simulink model "MBR_2025_09_29_Wassertank_nichtlinear_linear"  (R2024b)
settings: Solver=VariableStepAuto  StartTime=0.0  StopTime=10  RelTol=1e-3
settings Model: Creator=raroth  LastModifiedBy=marvincalmer

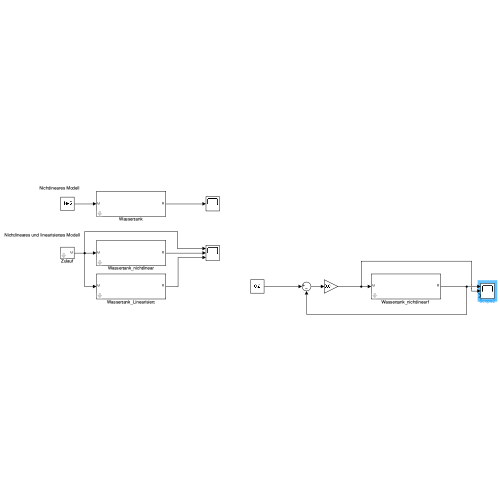
[thumbnail: Simulink's stored preview of the top-level diagram]
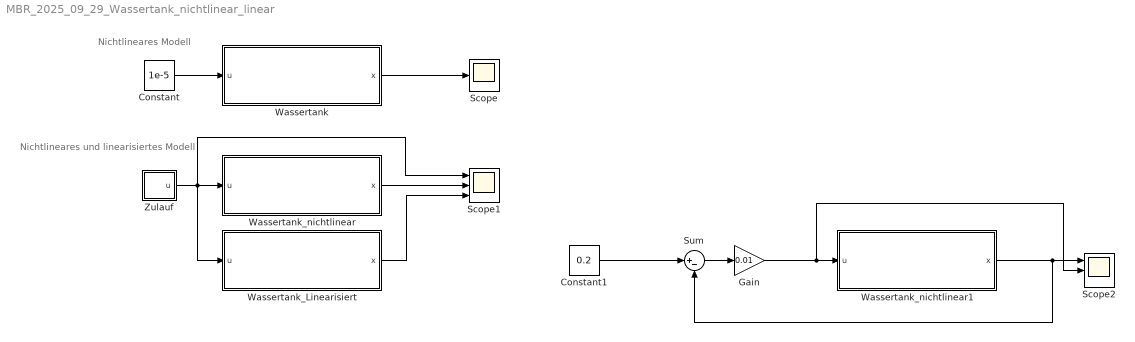
== system MBR_2025_09_29_Wassertank_nichtlinear_linear ==
  note: Nichtlineares Modell
  note: Nichtlineares und linearisiertes Modell
  Constant : Constant  Value=1e-5
  Constant1 : Constant  Value=0.2
  Gain : Gain  Gain=0.01
  Scope : Scope
  Scope1 : Scope  NumInputPorts=3
  Scope2 : Scope  NumInputPorts=3
  Sum : Sum  Inputs=|+-
  Wassertank : Subsystem  mask{dA=0.11, dc=4e-3, x0=0.1}
      mask prompts: dA "Durchmesser dA Grundfläche (m)"; dc "Durchmesser dc Ausflussquerschnitt (m)"; x0 "Anfangsfüllhöhe x0 (m)"
  Wassertank_Linearisiert : Subsystem  mask{dA=0.11, dc=4e-3, x0=0.1, xs=0.12}
      mask prompts: dA "Durchmesser dA Grundfläche (m)"; dc "Durchmesser dc Ausflussquerschnitt (m)"; x0 "Anfangsfüllhöhe x0 (m)"; xs "Linearisierungsstelle xs (m)"
  Wassertank_nichtlinear : Subsystem  mask{dA=0.11, dc=4e-3, x0=0.1}
      mask prompts: dA "Durchmesser dA Grundfläche (m)"; dc "Durchmesser dc Ausflussquerschnitt (m)"; x0 "Anfangsfüllhöhe x0 (m)"
  Wassertank_nichtlinear1 : Subsystem  mask{dA=0.11, dc=4e-3, x0=0.1}
      mask prompts: dA "Durchmesser dA Grundfläche (m)"; dc "Durchmesser dc Ausflussquerschnitt (m)"; x0 "Anfangsfüllhöhe x0 (m)"
  Zulauf : Subsystem  mask{dA=0.11, dc=4e-3, xs=0.13}
      mask prompts: dA "Durchmesser dA Grundfläche (m)"; dc "Durchmesser dc Ausflussquerschnitt (m)"; xs "Stationäre Füllhöhe xs (m)"
  wires:
  Constant/1 -> Wassertank/1(u)
  Wassertank/1(x) -> Scope/1
  Zulauf/1(u) -> Scope1/1, Wassertank_Linearisiert/1(u), Wassertank_nichtlinear/1(u)
  Wassertank_nichtlinear/1(x) -> Scope1/2
  Wassertank_Linearisiert/1(x) -> Scope1/3
  Wassertank_nichtlinear1/1(x) -> Sum/2, Scope2/1
  Constant1/1 -> Sum/1
  Sum/1 -> Gain/1
  Gain/1 -> Scope2/2, Wassertank_nichtlinear1/1(u)

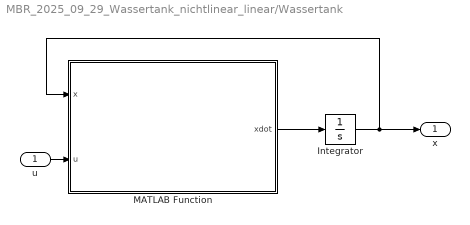
== system MBR_2025_09_29_Wassertank_nichtlinear_linear/Wassertank ==
  u : Inport
  Integrator : Integrator  InitialCondition=x0
  MATLAB Function : MATLAB Function  TreatAsAtomicUnit=on
  x : Outport
  wires:
  MATLAB Function/1(xdot) -> Integrator/1
  u/1 -> MATLAB Function/2(u)
  Integrator/1 -> x/1, MATLAB Function/1(x)

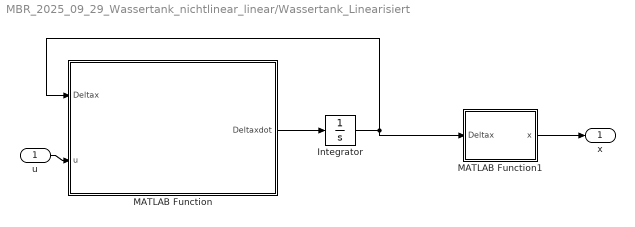
== system MBR_2025_09_29_Wassertank_nichtlinear_linear/Wassertank_Linearisiert ==
  u : Inport
  Integrator : Integrator  InitialCondition=x0-xs
  MATLAB Function : MATLAB Function  TreatAsAtomicUnit=on
  MATLAB Function1 : MATLAB Function  TreatAsAtomicUnit=on
  x : Outport
  wires:
  Integrator/1 -> MATLAB Function/1(Deltax), MATLAB Function1/1(Deltax)
  u/1 -> MATLAB Function/2(u)
  MATLAB Function/1(Deltaxdot) -> Integrator/1
  MATLAB Function1/1(x) -> x/1

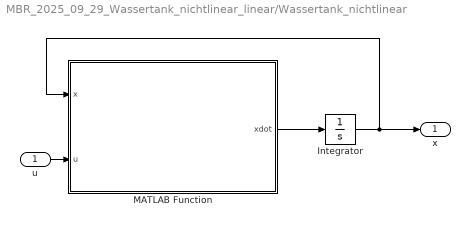
== system MBR_2025_09_29_Wassertank_nichtlinear_linear/Wassertank_nichtlinear ==
  u : Inport
  Integrator : Integrator  InitialCondition=x0
  MATLAB Function : MATLAB Function  TreatAsAtomicUnit=on
  x : Outport
  wires:
  MATLAB Function/1(xdot) -> Integrator/1
  u/1 -> MATLAB Function/2(u)
  Integrator/1 -> x/1, MATLAB Function/1(x)

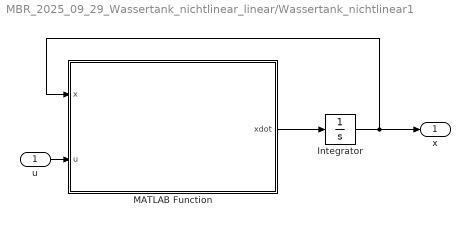
== system MBR_2025_09_29_Wassertank_nichtlinear_linear/Wassertank_nichtlinear1 ==
  u : Inport
  Integrator : Integrator  InitialCondition=x0
  MATLAB Function : MATLAB Function  TreatAsAtomicUnit=on
  x : Outport
  wires:
  MATLAB Function/1(xdot) -> Integrator/1
  u/1 -> MATLAB Function/2(u)
  Integrator/1 -> x/1, MATLAB Function/1(x)

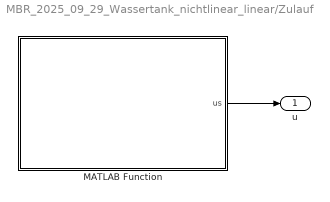
== system MBR_2025_09_29_Wassertank_nichtlinear_linear/Zulauf ==
  MATLAB Function : MATLAB Function  TreatAsAtomicUnit=on
  u : Outport
  wires:
  MATLAB Function/1(us) -> u/1

== matlab function MBR_2025_09_29_Wassertank_nichtlinear_linear/Wassertank_nichtlinear/MATLAB Function ==
  data: x input; u input; xdot output; dA parameter; dc parameter
function xdot = fcn(x, u, dA, dc)
% Parameter
  g  = 9.81;       % (m/s^2) Fallbeschleunigung
  A  = pi/4*dA^2;  % (m^2)   Behältergrundfläche
  Ac = pi/4*dc^2; % (m^2)   Ausflussquerschnittsfläche
% Modellparameter
  alpha = Ac/A*sqrt(2*g);
  beta  = 1/A;
% Volumenstrom
  Qdot = 0;
  if x>=0
    Qdot = alpha*sqrt(x);
  end
% Differentialgleichung
  xdot = beta*u-Qdot;
end

== matlab function MBR_2025_09_29_Wassertank_nichtlinear_linear/Wassertank/MATLAB Function ==
  data: x input; u input; xdot output; dA parameter; dc parameter
function xdot = fcn(x, u, dA, dc)
% Parameter
  g  = 9.81;       % (m/s^2) Fallbeschleunigung
  A  = pi/4*dA^2;  % (m^2)   Behältergrundfläche
  Ac = pi/4*dc^2; % (m^2)   Ausflussquerschnittsfläche
% Modellparameter
  alpha = Ac/A*sqrt(2*g);
  beta  = 1/A;
% Volumenstrom
  Qdot = 0;
  if x>=0
    Qdot = alpha*sqrt(x);
  end
% Differentialgleichung
  xdot = beta*u-Qdot;
end

== matlab function MBR_2025_09_29_Wassertank_nichtlinear_linear/Zulauf/MATLAB Function ==
  data: us output; dA parameter; dc parameter; xs parameter
function us = fcn(dA, dc, xs)
% Parameter
  g  = 9.81;       % (m/s^2) Fallbeschleunigung
  A  = pi/4*dA^2;  % (m^2)   Behältergrundfläche
  Ac = pi/4*dc^2; % (m^2)   Ausflussquerschnittsfläche
% Modellparameter
  alpha = Ac/A*sqrt(2*g);
  beta  = 1/A;
% Volumenstrom
  us = alpha/beta*sqrt(xs);
end

== matlab function MBR_2025_09_29_Wassertank_nichtlinear_linear/Wassertank_Linearisiert/MATLAB Function ==
  data: Deltax input; u input; Deltaxdot output; dA parameter; dc parameter; xs parameter
function Deltaxdot = fcn(Deltax, u, dA, dc, xs)
% Parameter
  g  = 9.81;       % (m/s^2) Fallbeschleunigung
  A  = pi/4*dA^2;  % (m^2)   Behältergrundfläche
  Ac = pi/4*dc^2; % (m^2)   Ausflussquerschnittsfläche
% Modellparameter
  alpha = Ac/A*sqrt(2*g);
  beta  = 1/A;
% Koeffizienten der linearisierten DGL
  a = alpha/(2*sqrt(xs));
  b = beta;
% Delta u
  us = alpha/beta*sqrt(xs);
  Deltau = u-us;
% Differentialgleichung
  Deltaxdot =-a*Deltax+ b*Deltau;
end

== matlab function MBR_2025_09_29_Wassertank_nichtlinear_linear/Wassertank_Linearisiert/MATLAB Function1 ==
  data: Deltax input; x output; xs parameter
function x = fcn(Deltax, xs)
  % Deltax = x-xs
    x = Deltax+xs;
end

== matlab function MBR_2025_09_29_Wassertank_nichtlinear_linear/Wassertank_nichtlinear1/MATLAB Function ==
  data: x input; u input; xdot output; dA parameter; dc parameter
function xdot = fcn(x, u, dA, dc)
% Parameter
  g  = 9.81;       % (m/s^2) Fallbeschleunigung
  A  = pi/4*dA^2;  % (m^2)   Behältergrundfläche
  Ac = pi/4*dc^2; % (m^2)   Ausflussquerschnittsfläche
% Modellparameter
  alpha = Ac/A*sqrt(2*g);
  beta  = 1/A;
% Volumenstrom
  Qdot = 0;
  if x>=0
    Qdot = alpha*sqrt(x);
  end
% Differentialgleichung
  xdot = beta*u-Qdot;
end
